simulink model "mDataStoreBlocksInsideLibraryLink"  (R2013b)
settings: Solver=FixedStepDiscrete  StartTime=0.0  StopTime=1  FixedStep=0.1  RelTol=1e-3
libraries: mDataStoreBlocks_library x2
settings Model: Creator=hungdang  LastModifiedBy=hungdang
settings OptimizationCC: InlineParams=on
settings DebuggingCC: InheritedTsInSrcMsg=none

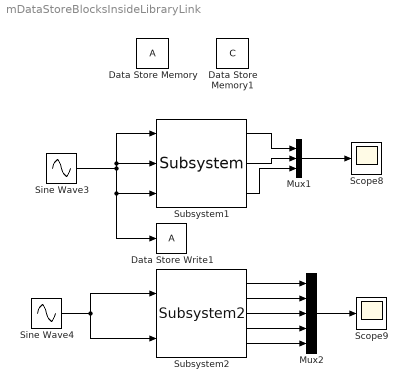
== system mDataStoreBlocksInsideLibraryLink ==
  Data Store Memory : DataStoreMemory  ReadBeforeWriteMsg=warning  WriteAfterWriteMsg=warning  WriteAfterReadMsg=warning
  Data Store Memory1 : DataStoreMemory  DataStoreName=C  ReadBeforeWriteMsg=warning  WriteAfterWriteMsg=warning  WriteAfterReadMsg=warning
  Data Store Write1 : DataStoreWrite
  Mux1 : Mux  Inputs=3
  Mux2 : Mux  Inputs=5
  Scope8 : Scope
      settings: SaveName=ScopeData8
  Scope9 : Scope
      settings: SaveName=ScopeData9
  Sine Wave3 : Sin  SampleTime=0.1
  Sine Wave4 : Sin  SampleTime=0
  Subsystem1 : mDataStoreBlocks_library/Subsystem
  Subsystem2 : mDataStoreBlocks_library/Subsystem2
  wires:
  Sine Wave3/1 -> Data Store Write1/1, Subsystem1/3, Subsystem1/2, Subsystem1/1
  Subsystem1/2 -> Mux1/2
  Subsystem1/1 -> Mux1/1
  Subsystem1/3 -> Mux1/3
  Mux1/1 -> Scope8/1
  Sine Wave4/1 -> Subsystem2/2, Subsystem2/1
  Subsystem2/3 -> Mux2/3
  Subsystem2/2 -> Mux2/2
  Subsystem2/4 -> Mux2/4
  Subsystem2/1 -> Mux2/1
  Mux2/1 -> Scope9/1
  Subsystem2/5 -> Mux2/5
